simulink model "ADRC_14a_mod1"  (R2014a)
settings: Solver=ode45  SolverMode=SingleTasking  StartTime=0.0  StopTime=50  RelTol=1e-3
model workspace (MAT data in the model file):
  b = Simulink.Parameter
  b.DataType = 'auto'
  b.Dimensions = [0 0]
  kp = Simulink.Parameter
  kp.DataType = 'auto'
  kp.Dimensions = [0 0]
settings Model: CovMetricSettings=dwe  CovHtmlReporting=off  covSaveCumulativeToWorkspaceVar=off  CovSaveSingleToWorkspaceVar=off  CovExternalEMLEnable=on  CovSFcnEnable=on  Creator=leony  LastModifiedBy=icaro
settings DataIOCC: LimitDataPoints=off  SaveFormat=StructureWithTime  ReturnWorkspaceOutputs=on
settings DebuggingCC: MergeDetectMultiDrivingBlocksExec=error  SolverPrmCheckMsg=none  FrameProcessingCompatibilityMsg=error  SFUnexpectedBacktrackingDiag=error  SFNoUnconditionalDefaultTransitionDiag=error
settings HardwareCC: ProdBitPerPointer=64  ProdLargestAtomicFloat=Float  ProdIntDivRoundTo=Zero  ProdEndianess=LittleEndian  ProdHWDeviceType=Specified
settings ModelReferenceCC: PropagateSignalLabelsOutOfModel=on
settings SFSimCC: SimUseLocalCustomCode=on
settings RTWCC: RTWUseLocalCustomCode=on
settings GRTTargetCC: TargetLangStandard=C99 (ISO)  GeneratePreprocessorConditionals=Use local settings

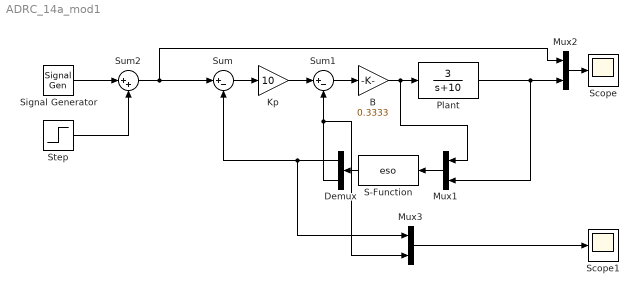
== system ADRC_14a_mod1 ==
  B : Gain  Gain=0.3333  ParamDataTypeStr=double
  Demux : Demux  Outputs=2
  Kp : Gain  Gain=10
  Mux1 : Mux  Inputs=2
  Mux2 : Mux  Inputs=2
  Mux3 : Mux  Inputs=2
  Plant : TransferFcn  Numerator=3  Denominator="[1  10]"
  S-Function : S-Function  FunctionName=eso  Parameters=b, kp  SFunctionDeploymentMode=off  EnableBusSupport=off
  Scope : Scope
      settings: TimeRange=auto  MaxDataPoints=5000  SaveToWorkspace=off  SaveName=ScopeData  YMin=-0.5  YMax=4.5  SampleTime=-1
  Scope1 : Scope
      settings: TimeRange=auto  MaxDataPoints=5000  SaveToWorkspace=off  YMin=-1.6665  YMax=14.9985  SampleTime=-1
  Signal Generator : SignalGenerator  WaveForm=square  Amplitude=2  Units=rad/sec
  Step : Step  Time=0  After=2  SampleTime=0
  Sum : Sum  Inputs=|+-
  Sum1 : Sum  Inputs=|+-
  Sum2 : Sum  Inputs=|++
  wires:
  Plant/1 -> Mux1/2, Mux2/2
  Mux1/1 -> S-Function/1
  S-Function/1 -> Demux/1
  Demux/1 -> Mux3/1, Sum/2
  Sum/1 -> Kp/1
  Kp/1 -> Sum1/1
  Demux/2 -> Mux3/2, Sum1/2
  Sum1/1 -> B/1
  B/1 -> Mux1/1, Plant/1
  Mux2/1 -> Scope/1
  Sum2/1 -> Mux2/1, Sum/1
  Step/1 -> Sum2/2
  Signal Generator/1 -> Sum2/1
  Mux3/1 -> Scope1/1
